simulink model "quadDyn"  (R2017a)
settings: Solver=ode45  StartTime=0.0  StopTime=100  FixedStep=1e-2  RelTol=1e-3  EnableMultiTasking=on
InitFcn:
  | m=0.285;
  | L=0.212;
  | g=9.807;
  | d=1;
  | Ix=5.136e-3;
  | Iy=5.136e-3;
  | Iz=1.016e-2;
  | alpha=diag([.42,.38,.5,.5,.3,.6]);
  | k=diag([2,3,1,6,5,30]);
  | lambda=diag([4.5,2,9.2,2.5,3.5,2]);
  | q=diag([0.4,0.4,.5,0.2,0.2,.1]);
  | beta=diag([0.2,0.2,0.2,0.38,0.3,0.2])
  | xi_0=[7;5;0;0;0;0];
  | xi_dot_0=[0;0;0;0;0;0];
  | xi_des=[0;0;8;5*pi/180;15*pi/180;10*pi/180]
  | xi_dot_des=[0;0;0;0;0;0];
  | xi_ddot_des=[0;0;0;0;0;0];
libraries: aerolibutil x2
settings Model: Creator=Ehsan  LastModifiedBy=Ehsan
settings SolverCC: AlgebraicLoopSolver=LineSearch
settings DataIOCC: LimitDataPoints=on  VisualizeSimOutput=off
settings OptimizationCC: LifeSpan=inf
settings DebuggingCC: AllowSymbolicDim=off  SFUnexpectedBacktrackingDiag=warning  SFNoUnconditionalDefaultTransitionDiag=warning  SFExecutionAtInitializationDiag=none
settings ModelReferenceCC: PropagateSignalLabelsOutOfModel=off
settings GRTTargetCC: TargetLangStandard=C89/C90 (ANSI)
settings ConfigComp: CovMetricSettings=dw  CovHtmlReporting=on  CovSaveCumulativeToWorkspaceVar=on  CovSaveSingleToWorkspaceVar=on  CovExternalEMLEnable=off

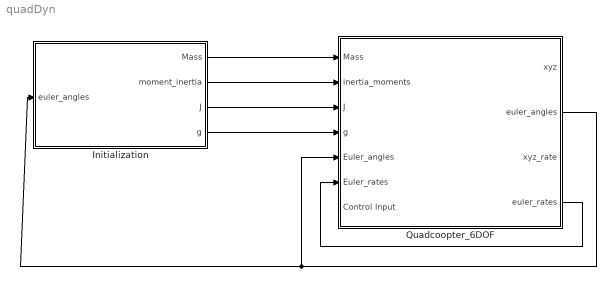
== system quadDyn ==
  Initialization : Subsystem
  Quadcoopter_6DOF : Subsystem
  wires:
  Quadcoopter_6DOF/2(euler_angles) -> Quadcoopter_6DOF/5(Euler_angles), Initialization/1(euler_angles)
  Quadcoopter_6DOF/4(euler_rates) -> Quadcoopter_6DOF/6(Euler_rates)
  Initialization/1(Mass) -> Quadcoopter_6DOF/1(Mass)
  Initialization/2(moment_inertia) -> Quadcoopter_6DOF/2(inertia_moments)
  Initialization/3(J) -> Quadcoopter_6DOF/3(J)
  Initialization/4(g) -> Quadcoopter_6DOF/4(g)

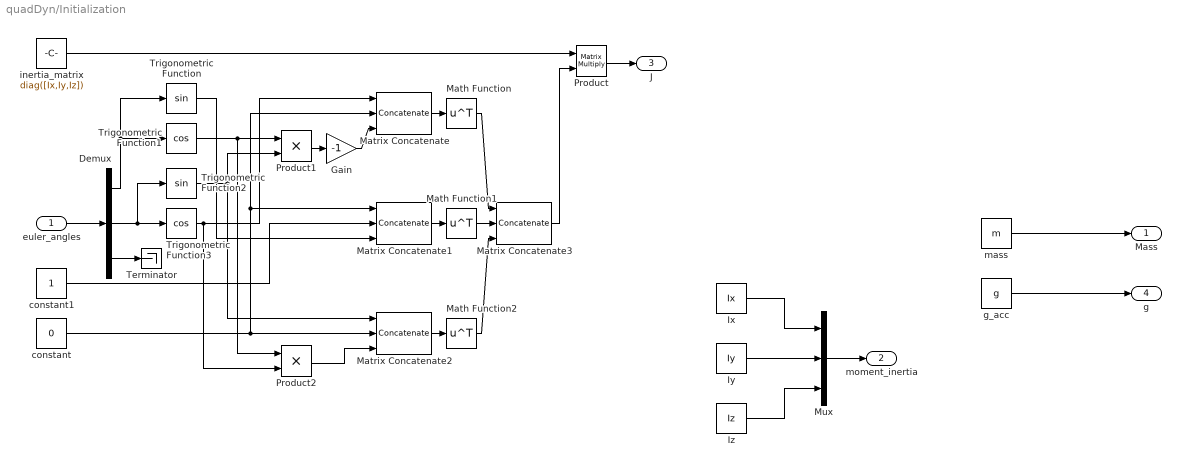
== system quadDyn/Initialization ==
  euler_angles : Inport
  Demux : Demux  Outputs=3
  Gain : Gain  Gain=-1
  Ix : Constant  Value=Ix
  Iy : Constant  Value=Iy
  Iz : Constant  Value=Iz
  Math Function : Math  Operator=transpose  SaturateOnIntegerOverflow=on
  Math Function1 : Math  Operator=transpose  SaturateOnIntegerOverflow=on
  Math Function2 : Math  Operator=transpose  SaturateOnIntegerOverflow=on
  Matrix Concatenate : Concatenate  NumInputs=3  ConcatenateDimension=2
  Matrix Concatenate1 : Concatenate  NumInputs=3  ConcatenateDimension=2
  Matrix Concatenate2 : Concatenate  NumInputs=3  ConcatenateDimension=2
  Matrix Concatenate3 : Concatenate  NumInputs=3  Mode=Multidimensional array
  Mux : Mux  Inputs=3
  Product : Product  Multiplication=Matrix(*)
  Product1 : Product
  Product2 : Product
  Terminator : Terminator
  Trigonometric Function : Trigonometry
  Trigonometric Function1 : Trigonometry  Operator=cos
  Trigonometric Function2 : Trigonometry
  Trigonometric Function3 : Trigonometry  Operator=cos
  constant : Constant  Value=0
  constant1 : Constant
  g_acc : Constant  Value=g
  inertia_matrix : Constant  Value=diag([Ix,Iy,Iz])
  mass : Constant  Value=m
  Mass : Outport
  moment_inertia : Outport  Port=2
  J : Outport  Port=3
  g : Outport  Port=4
  wires:
  mass/1 -> Mass/1
  Iy/1 -> Mux/2
  Ix/1 -> Mux/1
  Iz/1 -> Mux/3
  Mux/1 -> moment_inertia/1
  g_acc/1 -> g/1
  euler_angles/1 -> Demux/1
  Demux/3 -> Terminator/1
  Product/1 -> J/1
  inertia_matrix/1 -> Product/1
  Demux/1 -> Trigonometric Function/1, Trigonometric Function1/1
  Demux/2 -> Trigonometric Function3/1, Trigonometric Function2/1
  Trigonometric Function3/1 -> Product2/2, Matrix Concatenate/1
  constant/1 -> Matrix Concatenate1/1, Matrix Concatenate/2, Matrix Concatenate2/2
  Product1/1 -> Gain/1
  Trigonometric Function1/1 -> Product2/1, Product1/1
  Trigonometric Function2/1 -> Matrix Concatenate2/1, Product1/2
  Gain/1 -> Matrix Concatenate/3
  Trigonometric Function/1 -> Matrix Concatenate1/3
  constant1/1 -> Matrix Concatenate1/2
  Product2/1 -> Matrix Concatenate2/3
  Matrix Concatenate3/1 -> Product/2
  Matrix Concatenate/1 -> Math Function/1
  Matrix Concatenate1/1 -> Math Function1/1
  Math Function1/1 -> Matrix Concatenate3/2
  Matrix Concatenate2/1 -> Math Function2/1
  Math Function2/1 -> Matrix Concatenate3/3
  Math Function/1 -> Matrix Concatenate3/1

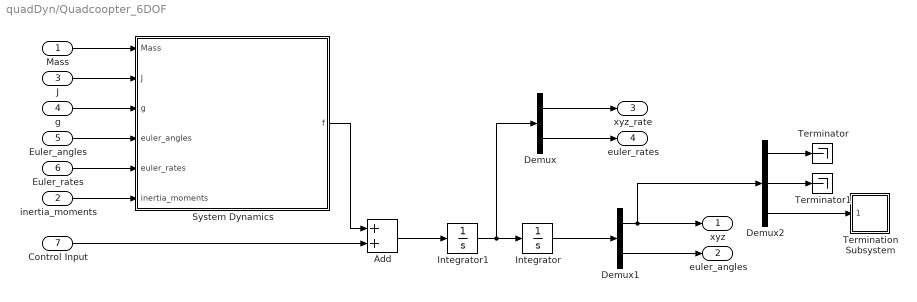
== system quadDyn/Quadcoopter_6DOF ==
  Mass : Inport
  inertia_moments : Inport  Port=2
  J : Inport  Port=3
  g : Inport  Port=4
  Euler_angles : Inport  Port=5
  Euler_rates : Inport  Port=6
  Control Input : Inport  Port=7
  Add : Sum
  Demux : Demux  Outputs=2
  Demux1 : Demux  Outputs=2
  Demux2 : Demux  Outputs=3
  Integrator : Integrator  InitialCondition=xi_0
  Integrator1 : Integrator  InitialCondition=xi_dot_0
  System Dynamics : Subsystem
  Termination Subsystem : Subsystem
  Terminator : Terminator
  Terminator1 : Terminator
  xyz : Outport
  euler_angles : Outport  Port=2
  xyz_rate : Outport  Port=3
  euler_rates : Outport  Port=4
  wires:
  Integrator1/1 -> Demux/1, Integrator/1
  Euler_rates/1 -> System Dynamics/5(euler_rates)
  System Dynamics/1(f) -> Add/1
  g/1 -> System Dynamics/3(g)
  J/1 -> System Dynamics/2(J)
  Mass/1 -> System Dynamics/1(Mass)
  Euler_angles/1 -> System Dynamics/4(euler_angles)
  inertia_moments/1 -> System Dynamics/6(inertia_moments)
  Integrator/1 -> Demux1/1
  Demux/2 -> euler_rates/1
  Demux1/1 -> Demux2/1, xyz/1
  Demux1/2 -> euler_angles/1
  Demux2/3 -> Termination Subsystem/1(Height)
  Demux/1 -> xyz_rate/1
  Demux2/1 -> Terminator/1
  Demux2/2 -> Terminator1/1
  Control Input/1 -> Add/2
  Add/1 -> Integrator1/1

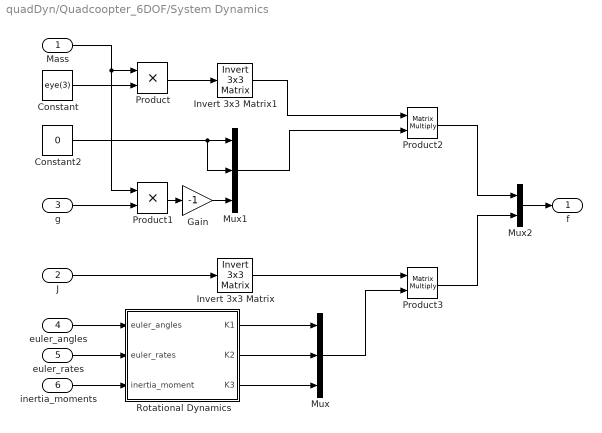
== system quadDyn/Quadcoopter_6DOF/System Dynamics ==
  Mass : Inport
  J : Inport  Port=2
  g : Inport  Port=3
  euler_angles : Inport  Port=4
  euler_rates : Inport  Port=5
  inertia_moments : Inport  Port=6
  Constant : Constant  Value=eye(3)
  Constant2 : Constant  Value=0
  Gain : Gain  Gain=-1
  Invert 3x3 Matrix : aerolibutil/Invert  3x3 Matrix
  Invert 3x3 Matrix1 : aerolibutil/Invert  3x3 Matrix
  Mux : Mux  Inputs=3
  Mux1 : Mux  Inputs=3
  Mux2 : Mux  Inputs=2
  Product : Product
  Product1 : Product
  Product2 : Product  Multiplication=Matrix(*)
  Product3 : Product  Multiplication=Matrix(*)
  Rotational Dynamics : Subsystem
  f : Outport
  wires:
  Rotational Dynamics/3(K3) -> Mux/3
  Constant/1 -> Product/2
  Mux2/1 -> f/1
  g/1 -> Product1/2
  Constant2/1 -> Mux1/2, Mux1/1
  Rotational Dynamics/1(K1) -> Mux/1
  Rotational Dynamics/2(K2) -> Mux/2
  Mass/1 -> Product1/1, Product/1
  euler_angles/1 -> Rotational Dynamics/1(euler_angles)
  euler_rates/1 -> Rotational Dynamics/2(euler_rates)
  inertia_moments/1 -> Rotational Dynamics/3(inertia_moment)
  Mux/1 -> Product3/2
  Product/1 -> Invert 3x3 Matrix1/1
  Mux1/1 -> Product2/2
  J/1 -> Invert 3x3 Matrix/1
  Invert 3x3 Matrix/1 -> Product3/1
  Invert 3x3 Matrix1/1 -> Product2/1
  Product2/1 -> Mux2/1
  Product3/1 -> Mux2/2
  Product1/1 -> Gain/1
  Gain/1 -> Mux1/3

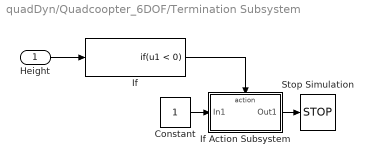
== system quadDyn/Quadcoopter_6DOF/Termination Subsystem ==
  Height : Inport
  Constant : Constant
  If : If  IfExpression=u1 < 0  ShowElse=off
  If Action Subsystem : Subsystem  TreatAsAtomicUnit=on
  Stop Simulation : Stop
  wires:
  If/1 -> If Action Subsystem/Action
  If Action Subsystem/1(Out1) -> Stop Simulation/1
  Constant/1 -> If Action Subsystem/1(In1)
  Height/1 -> If/1

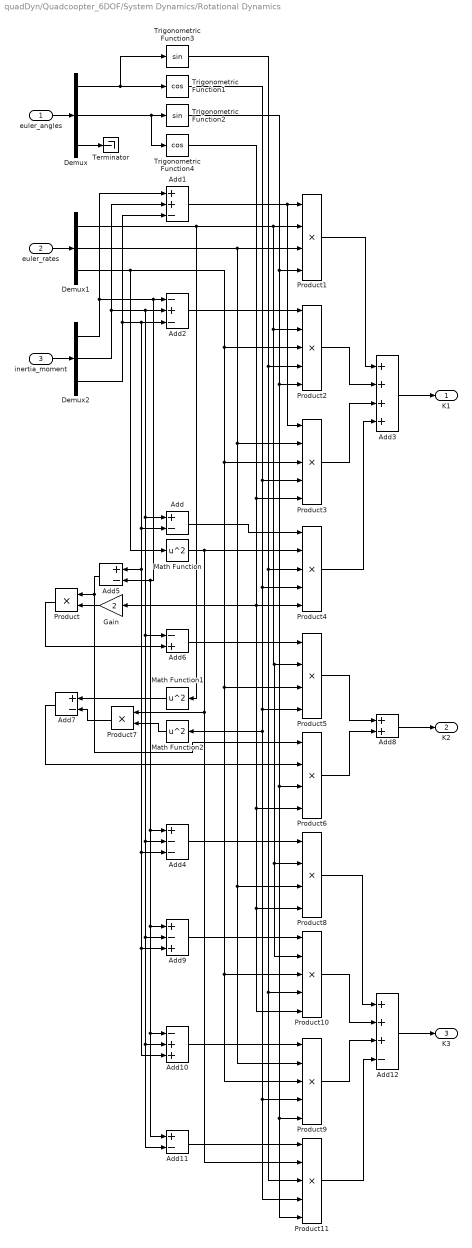
== system quadDyn/Quadcoopter_6DOF/System Dynamics/Rotational Dynamics ==
  euler_angles : Inport
  euler_rates : Inport  Port=2
  inertia_moment : Inport  Port=3
  Add{,5,7,11} (4 alike) : Sum  Inputs=+-
  Add1 : Sum  Inputs=++-
  Add10 : Sum  Inputs=-++
  Add12 : Sum  Inputs=+++-
  Add2 : Sum  Inputs=-+-
  Add3 : Sum  Inputs=++++
  Add4 : Sum  Inputs=+--
  Add6 : Sum  Inputs=-+
  Add8 : Sum
  Add9 : Sum  Inputs=+-+
  Demux : Demux  Outputs=3
  Demux1 : Demux  Outputs=3
  Demux2 : Demux  Outputs=3
  Gain : Gain  Gain=2
  Math Function : Math  Operator=square  SaturateOnIntegerOverflow=on
  Math Function1 : Math  Operator=square  SaturateOnIntegerOverflow=on
  Math Function2 : Math  Operator=square  SaturateOnIntegerOverflow=on
  Product : Product
  Product{1,5..6,8} (4 alike) : Product  Inputs=4
  Product{2..4,9..11} (6 alike) : Product  Inputs=5
  Product7 : Product
  Terminator : Terminator
  Trigonometric Function1 : Trigonometry  Operator=cos
  Trigonometric Function2 : Trigonometry
  Trigonometric Function3 : Trigonometry
  Trigonometric Function4 : Trigonometry  Operator=cos
  K1 : Outport
  K2 : Outport  Port=2
  K3 : Outport  Port=3
  wires:
  euler_angles/1 -> Demux/1
  euler_rates/1 -> Demux1/1
  inertia_moment/1 -> Demux2/1
  Demux/2 -> Trigonometric Function4/1, Trigonometric Function2/1
  Demux1/1 -> Math Function1/1, Product8/2, Product10/2, Product5/2, Product2/2, Product1/2
  Demux1/2 -> Product3/2, Product9/2, Product8/3, Product1/3
  Trigonometric Function2/1 -> Product11/5, Product9/5, Product6/3, Product2/5, Product1/4
  Add1/1 -> Product3/1, Product1/1
  Demux2/1 -> Add11/1, Add10/1, Add9/1, Add4/1, Add5/2, Add2/1, Add1/1
  Demux2/2 -> Add11/2, Add10/2, Add9/2, Add4/2, Add6/1, Add/1, Add2/2, Add1/2
  Demux2/3 -> Add2/3, Add5/1, Add10/3, Add9/3, Add4/3, Add/2, Add1/3
  Demux/1 -> Trigonometric Function3/1, Trigonometric Function1/1
  Trigonometric Function3/1 -> Product11/3, Product10/4, Product4/3, Product2/4
  Demux1/3 -> Math Function/1, Product9/3, Product10/3, Product5/3, Product3/3, Product2/3
  Add2/1 -> Product2/1
  Trigonometric Function4/1 -> Gain/1, Product10/5, Product8/4, Product6/4, Product4/5, Product3/5
  Trigonometric Function1/1 -> Product5/4, Math Function2/1, Product11/4, Product9/4, Product4/4, Product3/4
  Math Function/1 -> Product11/2, Product7/1, Product4/2
  Add/1 -> Product4/1
  Product2/1 -> Add3/2
  Product3/1 -> Add3/3
  Product1/1 -> Add3/1
  Product4/1 -> Add3/4
  Add3/1 -> K1/1
  Add5/1 -> Product6/1, Product/1
  Gain/1 -> Product/2
  Add6/1 -> Product5/1
  Product/1 -> Add6/2
  Product7/1 -> Add7/2
  Add7/1 -> Product6/2
  Math Function2/1 -> Product7/2
  Add8/1 -> K2/1
  Product5/1 -> Add8/1
  Product6/1 -> Add8/2
  Add4/1 -> Product8/1
  Add9/1 -> Product10/1
  Add10/1 -> Product9/1
  Add11/1 -> Product11/1
  Product9/1 -> Add12/3
  Product10/1 -> Add12/2
  Product11/1 -> Add12/4
  Product8/1 -> Add12/1
  Add12/1 -> K3/1
  Demux/3 -> Terminator/1
  Math Function1/1 -> Add7/1

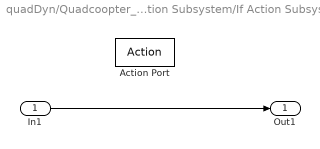
== system quadDyn/Quadcoopter_6DOF/Termination Subsystem/If Action Subsystem ==
  In1 : Inport
  Action Port : ActionPort  ActionType=then
  Out1 : Outport
  wires:
  In1/1 -> Out1/1
